simulink model "V2V"  (R2023a)
settings: Solver=FixedStepDiscrete  StartTime=0.0  StopTime=10  FixedStep=0.1  RelTol=1e-3
undefined symbols (not defined in the file): samp_time
(part 2 of 2)

== system V2V/Subsystem28/Subsystem ==
  x1 : Inport
  In2 : Inport  Port=2
  In3 : Inport  Port=3
  x2 : Inport  Port=4
  r : Inport  Port=5
  MATLAB Function : MATLAB Function  TreatAsAtomicUnit=on  SystemSampleTime=0.1
  Switch : Switch  Criteria=u2 > Threshold  SaturateOnIntegerOverflow=off  InputSameDT=off
  Out1 : Outport
  wires:
  x2/1 -> MATLAB Function/2(x2)
  x1/1 -> MATLAB Function/1(x1)
  Switch/1 -> Out1/1
  In2/1 -> Switch/1
  In3/1 -> Switch/3
  MATLAB Function/1(y) -> Switch/2
  r/1 -> MATLAB Function/3(r)

== system V2V/Subsystem30/Subsystem ==
  x1 : Inport
  In2 : Inport  Port=2
  In3 : Inport  Port=3
  x2 : Inport  Port=4
  r : Inport  Port=5
  MATLAB Function : MATLAB Function  TreatAsAtomicUnit=on  SystemSampleTime=0.1
  Switch : Switch  Criteria=u2 > Threshold  SaturateOnIntegerOverflow=off  InputSameDT=off
  Out1 : Outport
  wires:
  x2/1 -> MATLAB Function/2(x2)
  x1/1 -> MATLAB Function/1(x1)
  Switch/1 -> Out1/1
  In2/1 -> Switch/1
  In3/1 -> Switch/3
  MATLAB Function/1(y) -> Switch/2
  r/1 -> MATLAB Function/3(r)

== system V2V/Subsystem31/Subsystem ==
  x1 : Inport
  In2 : Inport  Port=2
  In3 : Inport  Port=3
  x2 : Inport  Port=4
  r : Inport  Port=5
  MATLAB Function : MATLAB Function  TreatAsAtomicUnit=on  SystemSampleTime=0.1
  Switch : Switch  Criteria=u2 > Threshold  SaturateOnIntegerOverflow=off  InputSameDT=off
  Out1 : Outport
  wires:
  x2/1 -> MATLAB Function/2(x2)
  x1/1 -> MATLAB Function/1(x1)
  Switch/1 -> Out1/1
  In2/1 -> Switch/1
  In3/1 -> Switch/3
  MATLAB Function/1(y) -> Switch/2
  r/1 -> MATLAB Function/3(r)

== system V2V/Subsystem33/Subsystem ==
  x1 : Inport
  In2 : Inport  Port=2
  In3 : Inport  Port=3
  x2 : Inport  Port=4
  r : Inport  Port=5
  MATLAB Function : MATLAB Function  TreatAsAtomicUnit=on  SystemSampleTime=0.1
  Switch : Switch  Criteria=u2 > Threshold  SaturateOnIntegerOverflow=off  InputSameDT=off
  Out1 : Outport
  wires:
  x2/1 -> MATLAB Function/2(x2)
  x1/1 -> MATLAB Function/1(x1)
  Switch/1 -> Out1/1
  In2/1 -> Switch/1
  In3/1 -> Switch/3
  MATLAB Function/1(y) -> Switch/2
  r/1 -> MATLAB Function/3(r)

== system V2V/Subsystem34/Subsystem ==
  x1 : Inport
  In2 : Inport  Port=2
  In3 : Inport  Port=3
  x2 : Inport  Port=4
  r : Inport  Port=5
  MATLAB Function : MATLAB Function  TreatAsAtomicUnit=on  SystemSampleTime=0.1
  Switch : Switch  Criteria=u2 > Threshold  SaturateOnIntegerOverflow=off  InputSameDT=off
  Out1 : Outport
  wires:
  x2/1 -> MATLAB Function/2(x2)
  x1/1 -> MATLAB Function/1(x1)
  Switch/1 -> Out1/1
  In2/1 -> Switch/1
  In3/1 -> Switch/3
  MATLAB Function/1(y) -> Switch/2
  r/1 -> MATLAB Function/3(r)

== system V2V/Subsystem36/Subsystem ==
  x1 : Inport
  In2 : Inport  Port=2
  In3 : Inport  Port=3
  x2 : Inport  Port=4
  r : Inport  Port=5
  MATLAB Function : MATLAB Function  TreatAsAtomicUnit=on  SystemSampleTime=0.1
  Switch : Switch  Criteria=u2 > Threshold  SaturateOnIntegerOverflow=off  InputSameDT=off
  Out1 : Outport
  wires:
  x2/1 -> MATLAB Function/2(x2)
  x1/1 -> MATLAB Function/1(x1)
  Switch/1 -> Out1/1
  In2/1 -> Switch/1
  In3/1 -> Switch/3
  MATLAB Function/1(y) -> Switch/2
  r/1 -> MATLAB Function/3(r)

== system V2V/Subsystem37/Subsystem ==
  x1 : Inport
  In2 : Inport  Port=2
  In3 : Inport  Port=3
  x2 : Inport  Port=4
  r : Inport  Port=5
  MATLAB Function : MATLAB Function  TreatAsAtomicUnit=on  SystemSampleTime=0.1
  Switch : Switch  Criteria=u2 > Threshold  SaturateOnIntegerOverflow=off  InputSameDT=off
  Out1 : Outport
  wires:
  x2/1 -> MATLAB Function/2(x2)
  x1/1 -> MATLAB Function/1(x1)
  Switch/1 -> Out1/1
  In2/1 -> Switch/1
  In3/1 -> Switch/3
  MATLAB Function/1(y) -> Switch/2
  r/1 -> MATLAB Function/3(r)

== system V2V/Subsystem39/Subsystem ==
  x1 : Inport
  In2 : Inport  Port=2
  In3 : Inport  Port=3
  x2 : Inport  Port=4
  r : Inport  Port=5
  MATLAB Function : MATLAB Function  TreatAsAtomicUnit=on  SystemSampleTime=0.1
  Switch : Switch  Criteria=u2 > Threshold  SaturateOnIntegerOverflow=off  InputSameDT=off
  Out1 : Outport
  wires:
  x2/1 -> MATLAB Function/2(x2)
  x1/1 -> MATLAB Function/1(x1)
  Switch/1 -> Out1/1
  In2/1 -> Switch/1
  In3/1 -> Switch/3
  MATLAB Function/1(y) -> Switch/2
  r/1 -> MATLAB Function/3(r)

== system V2V/Subsystem40/Subsystem ==
  x1 : Inport
  In2 : Inport  Port=2
  In3 : Inport  Port=3
  x2 : Inport  Port=4
  r : Inport  Port=5
  MATLAB Function : MATLAB Function  TreatAsAtomicUnit=on  SystemSampleTime=0.1
  Switch : Switch  Criteria=u2 > Threshold  SaturateOnIntegerOverflow=off  InputSameDT=off
  Out1 : Outport
  wires:
  x2/1 -> MATLAB Function/2(x2)
  x1/1 -> MATLAB Function/1(x1)
  Switch/1 -> Out1/1
  In2/1 -> Switch/1
  In3/1 -> Switch/3
  MATLAB Function/1(y) -> Switch/2
  r/1 -> MATLAB Function/3(r)

== system V2V/Subsystem42/Subsystem ==
  x1 : Inport
  In2 : Inport  Port=2
  In3 : Inport  Port=3
  x2 : Inport  Port=4
  r : Inport  Port=5
  MATLAB Function : MATLAB Function  TreatAsAtomicUnit=on  SystemSampleTime=0.1
  Switch : Switch  Criteria=u2 > Threshold  SaturateOnIntegerOverflow=off  InputSameDT=off
  Out1 : Outport
  wires:
  x2/1 -> MATLAB Function/2(x2)
  x1/1 -> MATLAB Function/1(x1)
  Switch/1 -> Out1/1
  In2/1 -> Switch/1
  In3/1 -> Switch/3
  MATLAB Function/1(y) -> Switch/2
  r/1 -> MATLAB Function/3(r)

== system V2V/Subsystem43/Subsystem ==
  x1 : Inport
  In2 : Inport  Port=2
  In3 : Inport  Port=3
  x2 : Inport  Port=4
  r : Inport  Port=5
  MATLAB Function : MATLAB Function  TreatAsAtomicUnit=on  SystemSampleTime=0.1
  Switch : Switch  Criteria=u2 > Threshold  SaturateOnIntegerOverflow=off  InputSameDT=off
  Out1 : Outport
  wires:
  x2/1 -> MATLAB Function/2(x2)
  x1/1 -> MATLAB Function/1(x1)
  Switch/1 -> Out1/1
  In2/1 -> Switch/1
  In3/1 -> Switch/3
  MATLAB Function/1(y) -> Switch/2
  r/1 -> MATLAB Function/3(r)

== system V2V/Subsystem45/Subsystem ==
  x1 : Inport
  In2 : Inport  Port=2
  In3 : Inport  Port=3
  x2 : Inport  Port=4
  r : Inport  Port=5
  MATLAB Function : MATLAB Function  TreatAsAtomicUnit=on  SystemSampleTime=0.1
  Switch : Switch  Criteria=u2 > Threshold  SaturateOnIntegerOverflow=off  InputSameDT=off
  Out1 : Outport
  wires:
  x2/1 -> MATLAB Function/2(x2)
  x1/1 -> MATLAB Function/1(x1)
  Switch/1 -> Out1/1
  In2/1 -> Switch/1
  In3/1 -> Switch/3
  MATLAB Function/1(y) -> Switch/2
  r/1 -> MATLAB Function/3(r)

== system V2V/Subsystem46/Subsystem ==
  x1 : Inport
  In2 : Inport  Port=2
  In3 : Inport  Port=3
  x2 : Inport  Port=4
  r : Inport  Port=5
  MATLAB Function : MATLAB Function  TreatAsAtomicUnit=on  SystemSampleTime=0.1
  Switch : Switch  Criteria=u2 > Threshold  SaturateOnIntegerOverflow=off  InputSameDT=off
  Out1 : Outport
  wires:
  x2/1 -> MATLAB Function/2(x2)
  x1/1 -> MATLAB Function/1(x1)
  Switch/1 -> Out1/1
  In2/1 -> Switch/1
  In3/1 -> Switch/3
  MATLAB Function/1(y) -> Switch/2
  r/1 -> MATLAB Function/3(r)

== system V2V/Subsystem48/Subsystem ==
  x1 : Inport
  In2 : Inport  Port=2
  In3 : Inport  Port=3
  x2 : Inport  Port=4
  r : Inport  Port=5
  MATLAB Function : MATLAB Function  TreatAsAtomicUnit=on  SystemSampleTime=0.1
  Switch : Switch  Criteria=u2 > Threshold  SaturateOnIntegerOverflow=off  InputSameDT=off
  Out1 : Outport
  wires:
  x2/1 -> MATLAB Function/2(x2)
  x1/1 -> MATLAB Function/1(x1)
  Switch/1 -> Out1/1
  In2/1 -> Switch/1
  In3/1 -> Switch/3
  MATLAB Function/1(y) -> Switch/2
  r/1 -> MATLAB Function/3(r)

== system V2V/Subsystem49/Subsystem ==
  x1 : Inport
  In2 : Inport  Port=2
  In3 : Inport  Port=3
  x2 : Inport  Port=4
  r : Inport  Port=5
  MATLAB Function : MATLAB Function  TreatAsAtomicUnit=on  SystemSampleTime=0.1
  Switch : Switch  Criteria=u2 > Threshold  SaturateOnIntegerOverflow=off  InputSameDT=off
  Out1 : Outport
  wires:
  x2/1 -> MATLAB Function/2(x2)
  x1/1 -> MATLAB Function/1(x1)
  Switch/1 -> Out1/1
  In2/1 -> Switch/1
  In3/1 -> Switch/3
  MATLAB Function/1(y) -> Switch/2
  r/1 -> MATLAB Function/3(r)

== system V2V/Subsystem5/Subsystem ==
  x1 : Inport
  In2 : Inport  Port=2
  In3 : Inport  Port=3
  x2 : Inport  Port=4
  r : Inport  Port=5
  MATLAB Function : MATLAB Function  TreatAsAtomicUnit=on  SystemSampleTime=0.1
  Switch : Switch  Criteria=u2 > Threshold  SaturateOnIntegerOverflow=off  InputSameDT=off
  Out1 : Outport
  wires:
  x2/1 -> MATLAB Function/2(x2)
  x1/1 -> MATLAB Function/1(x1)
  Switch/1 -> Out1/1
  In2/1 -> Switch/1
  In3/1 -> Switch/3
  MATLAB Function/1(y) -> Switch/2
  r/1 -> MATLAB Function/3(r)

== system V2V/Subsystem51/Subsystem ==
  x1 : Inport
  In2 : Inport  Port=2
  In3 : Inport  Port=3
  x2 : Inport  Port=4
  r : Inport  Port=5
  MATLAB Function : MATLAB Function  TreatAsAtomicUnit=on  SystemSampleTime=0.1
  Switch : Switch  Criteria=u2 > Threshold  SaturateOnIntegerOverflow=off  InputSameDT=off
  Out1 : Outport
  wires:
  x2/1 -> MATLAB Function/2(x2)
  x1/1 -> MATLAB Function/1(x1)
  Switch/1 -> Out1/1
  In2/1 -> Switch/1
  In3/1 -> Switch/3
  MATLAB Function/1(y) -> Switch/2
  r/1 -> MATLAB Function/3(r)

== system V2V/Subsystem52/Subsystem ==
  x1 : Inport
  In2 : Inport  Port=2
  In3 : Inport  Port=3
  x2 : Inport  Port=4
  r : Inport  Port=5
  MATLAB Function : MATLAB Function  TreatAsAtomicUnit=on  SystemSampleTime=0.1
  Switch : Switch  Criteria=u2 > Threshold  SaturateOnIntegerOverflow=off  InputSameDT=off
  Out1 : Outport
  wires:
  x2/1 -> MATLAB Function/2(x2)
  x1/1 -> MATLAB Function/1(x1)
  Switch/1 -> Out1/1
  In2/1 -> Switch/1
  In3/1 -> Switch/3
  MATLAB Function/1(y) -> Switch/2
  r/1 -> MATLAB Function/3(r)

== system V2V/Subsystem54/Subsystem ==
  x1 : Inport
  In2 : Inport  Port=2
  In3 : Inport  Port=3
  x2 : Inport  Port=4
  r : Inport  Port=5
  MATLAB Function : MATLAB Function  TreatAsAtomicUnit=on  SystemSampleTime=0.1
  Switch : Switch  Criteria=u2 > Threshold  SaturateOnIntegerOverflow=off  InputSameDT=off
  Out1 : Outport
  wires:
  x2/1 -> MATLAB Function/2(x2)
  x1/1 -> MATLAB Function/1(x1)
  Switch/1 -> Out1/1
  In2/1 -> Switch/1
  In3/1 -> Switch/3
  MATLAB Function/1(y) -> Switch/2
  r/1 -> MATLAB Function/3(r)

== system V2V/Subsystem55/Subsystem ==
  x1 : Inport
  In2 : Inport  Port=2
  In3 : Inport  Port=3
  x2 : Inport  Port=4
  r : Inport  Port=5
  MATLAB Function : MATLAB Function  TreatAsAtomicUnit=on  SystemSampleTime=0.1
  Switch : Switch  Criteria=u2 > Threshold  SaturateOnIntegerOverflow=off  InputSameDT=off
  Out1 : Outport
  wires:
  x2/1 -> MATLAB Function/2(x2)
  x1/1 -> MATLAB Function/1(x1)
  Switch/1 -> Out1/1
  In2/1 -> Switch/1
  In3/1 -> Switch/3
  MATLAB Function/1(y) -> Switch/2
  r/1 -> MATLAB Function/3(r)

== system V2V/Subsystem6/Subsystem ==
  x1 : Inport
  In2 : Inport  Port=2
  In3 : Inport  Port=3
  x2 : Inport  Port=4
  r : Inport  Port=5
  MATLAB Function : MATLAB Function  TreatAsAtomicUnit=on  SystemSampleTime=0.1
  Switch : Switch  Criteria=u2 > Threshold  SaturateOnIntegerOverflow=off  InputSameDT=off
  Out1 : Outport
  wires:
  x2/1 -> MATLAB Function/2(x2)
  x1/1 -> MATLAB Function/1(x1)
  Switch/1 -> Out1/1
  In2/1 -> Switch/1
  In3/1 -> Switch/3
  MATLAB Function/1(y) -> Switch/2
  r/1 -> MATLAB Function/3(r)

== system V2V/Subsystem7/Subsystem ==
  x1 : Inport
  In2 : Inport  Port=2
  In3 : Inport  Port=3
  x2 : Inport  Port=4
  r : Inport  Port=5
  MATLAB Function : MATLAB Function  TreatAsAtomicUnit=on  SystemSampleTime=0.1
  Switch : Switch  Criteria=u2 > Threshold  SaturateOnIntegerOverflow=off  InputSameDT=off
  Out1 : Outport
  wires:
  x2/1 -> MATLAB Function/2(x2)
  x1/1 -> MATLAB Function/1(x1)
  Switch/1 -> Out1/1
  In2/1 -> Switch/1
  In3/1 -> Switch/3
  MATLAB Function/1(y) -> Switch/2
  r/1 -> MATLAB Function/3(r)

== matlab function V2V/MATLAB Function ==
  data: delay_txL output; delay_tx2 output; delay_tx3 output; delay_tx4 output; delay_tx5 output; delay_tx6 output; delay_tx7 output; delay_tx8 output; delay_tx9 output; delay_tx10 output; delay_tx11 output; delay_tx12 output; delay_tx13 output; delay_tx14 output; delay_tx15 output; delay_tx16 output; delay_tx17 output; delay_tx18 output; delay_tx19 output; p_rx_L_2 output; p_rx_L_3 output; p_rx_L_4 output; p_rx_L_5 output; p_rx_L_6 output; p_rx_L_7 output; p_rx_L_8 output; p_rx_L_9 output; p_rx_L_10 output; p_rx_L_11 output; p_rx_L_12 output; p_rx_L_13 output; p_rx_L_14 output; p_rx_L_15 output; p_rx_L_16 output; p_rx_L_17 output; p_rx_L_18 output; p_rx_L_19 output; p_rx_L_20 output; p_rx_2_3 output; p_rx_3_4 output; p_rx_4_5 output; p_rx_5_6 output; p_rx_6_7 output; p_rx_7_8 output; p_rx_8_9 output; p_rx_9_10 output; p_rx_10_11 output; p_rx_11_12 output; p_rx_12_13 output; p_rx_13_14 output; p_rx_14_15 output; p_rx_15_16 output; p_rx_16_17 output; p_rx_17_18 output; p_rx_18_19 output; p_rx_19_20 output; data input
function [delay_txL,delay_tx2,delay_tx3,delay_tx4,delay_tx5,delay_tx6,delay_tx7,delay_tx8,delay_tx9,delay_tx10,delay_tx11,delay_tx12,delay_tx13,delay_tx14,delay_tx15,delay_tx16,delay_tx17,delay_tx18,delay_tx19,...
        p_rx_L_2,p_rx_L_3,p_rx_L_4,p_rx_L_5,p_rx_L_6,p_rx_L_7,p_rx_L_8,p_rx_L_9,p_rx_L_10,p_rx_L_11,p_rx_L_12,p_rx_L_13,p_rx_L_14,p_rx_L_15,p_rx_L_16,p_rx_L_17,p_rx_L_18,p_rx_L_19,p_rx_L_20,...
        p_rx_2_3,p_rx_3_4,p_rx_4_5,p_rx_5_6,p_rx_6_7,p_rx_7_8,p_rx_8_9,p_rx_9_10,p_rx_10_11,p_rx_11_12,p_rx_12_13,p_rx_13_14,p_rx_14_15,p_rx_15_16,p_rx_16_17,p_rx_17_18,p_rx_18_19,p_rx_19_20] = fcn(data)
delay_txL = ceil(exprnd(20));
delay_tx2 = ceil(exprnd(20));
delay_tx3 = ceil(exprnd(20));
delay_tx4 = ceil(exprnd(20));
delay_tx5 = ceil(exprnd(20));
delay_tx6 = ceil(exprnd(20));
delay_tx7 = ceil(exprnd(20));
delay_tx8 = ceil(exprnd(20));
delay_tx9 = ceil(exprnd(20));
delay_tx10 = ceil(exprnd(20));
delay_tx11 = ceil(exprnd(20));
delay_tx12 = ceil(exprnd(20));
delay_tx13 = ceil(exprnd(20));
delay_tx14 = ceil(exprnd(20));
delay_tx15 = ceil(exprnd(20));
delay_tx16 = ceil(exprnd(20));
delay_tx17 = ceil(exprnd(20));
delay_tx18 = ceil(exprnd(20));
delay_tx19 = ceil(exprnd(20));

p_rx_L_2 = rand;
p_rx_L_3 = rand;
p_rx_L_4 = rand;
p_rx_L_5 = rand;
p_rx_L_6 = rand;
p_rx_L_7 = rand;
p_rx_L_8 = rand;
p_rx_L_9 = rand;
p_rx_L_10 = rand;
p_rx_L_11 = rand;
p_rx_L_12 = rand;
p_rx_L_13 = rand;
p_rx_L_14 = rand;
p_rx_L_15 = rand;
p_rx_L_16 = rand;
p_rx_L_17 = rand;
p_rx_L_18 = rand;
p_rx_L_19 = rand;
p_rx_L_20 = rand;

p_rx_2_3 = rand;
p_rx_3_4 = rand;
p_rx_4_5 = rand;
p_rx_5_6 = rand;
p_rx_6_7 = rand;
p_rx_7_8 = rand;
p_rx_8_9 = rand;
p_rx_9_10 = rand;
p_rx_10_11 = rand;
p_rx_11_12 = rand;
p_rx_12_13 = rand;
p_rx_13_14 = rand;
p_rx_14_15 = rand;
p_rx_15_16 = rand;
p_rx_16_17 = rand;
p_rx_17_18 = rand;
p_rx_18_19 = rand;
p_rx_19_20 = rand;
end

== matlab function V2V/Subsystem10/Subsystem/MATLAB Function ==
  data: x1 input; y output; x2 input; r input
function y = fcn(x1,x2,r)
    PDR = model80211p(0.12,25,23,190,6e6,x1-x2);

    y = r < PDR;
end

== matlab function V2V/Subsystem11/Subsystem/MATLAB Function ==
  data: x1 input; y output; x2 input; r input
function y = fcn(x1,x2,r)
    PDR = model80211p(0.12,25,23,190,6e6,x1-x2);

    y = r < PDR;
end

== matlab function V2V/Subsystem12/Subsystem/MATLAB Function ==
  data: x1 input; y output; x2 input; r input
function y = fcn(x1,x2,r)
    PDR = model80211p(0.12,25,23,190,6e6,x1-x2);

    y = r < PDR;
end

== matlab function V2V/Subsystem5/Subsystem/MATLAB Function ==
  data: x1 input; y output; x2 input; r input
function y = fcn(x1,x2,r)
    PDR = model80211p(0.12,25,23,190,6e6,x1-x2);

    y = r < PDR;
end

== matlab function V2V/Subsystem13/Subsystem/MATLAB Function ==
  data: x1 input; y output; x2 input; r input
function y = fcn(x1,x2,r)
    PDR = model80211p(0.12,25,23,190,6e6,x1-x2);

    y = r < PDR;
end

== matlab function V2V/Subsystem15/Subsystem/MATLAB Function ==
  data: x1 input; y output; x2 input; r input
function y = fcn(x1,x2,r)
    PDR = model80211p(0.12,25,23,190,6e6,x1-x2);

    y = r < PDR;
end

== matlab function V2V/Subsystem16/Subsystem/MATLAB Function ==
  data: x1 input; y output; x2 input; r input
function y = fcn(x1,x2,r)
    PDR = model80211p(0.12,25,23,190,6e6,x1-x2);

    y = r < PDR;
end

== matlab function V2V/Subsystem18/Subsystem/MATLAB Function ==
  data: x1 input; y output; x2 input; r input
function y = fcn(x1,x2,r)
    PDR = model80211p(0.12,25,23,190,6e6,x1-x2);

    y = r < PDR;
end

== matlab function V2V/Subsystem19/Subsystem/MATLAB Function ==
  data: x1 input; y output; x2 input; r input
function y = fcn(x1,x2,r)
    PDR = model80211p(0.12,25,23,190,6e6,x1-x2);

    y = r < PDR;
end

== matlab function V2V/Subsystem21/Subsystem/MATLAB Function ==
  data: x1 input; y output; x2 input; r input
function y = fcn(x1,x2,r)
    PDR = model80211p(0.12,25,23,190,6e6,x1-x2);

    y = r < PDR;
end

== matlab function V2V/Subsystem22/Subsystem/MATLAB Function ==
  data: x1 input; y output; x2 input; r input
function y = fcn(x1,x2,r)
    PDR = model80211p(0.12,25,23,190,6e6,x1-x2);

    y = r < PDR;
end

== matlab function V2V/Subsystem24/Subsystem/MATLAB Function ==
  data: x1 input; y output; x2 input; r input
function y = fcn(x1,x2,r)
    PDR = model80211p(0.12,25,23,190,6e6,x1-x2);

    y = r < PDR;
end

== matlab function V2V/Subsystem25/Subsystem/MATLAB Function ==
  data: x1 input; y output; x2 input; r input
function y = fcn(x1,x2,r)
    PDR = model80211p(0.12,25,23,190,6e6,x1-x2);

    y = r < PDR;
end

== matlab function V2V/Subsystem27/Subsystem/MATLAB Function ==
  data: x1 input; y output; x2 input; r input
function y = fcn(x1,x2,r)
    PDR = model80211p(0.12,25,23,190,6e6,x1-x2);

    y = r < PDR;
end

== matlab function V2V/Subsystem28/Subsystem/MATLAB Function ==
  data: x1 input; y output; x2 input; r input
function y = fcn(x1,x2,r)
    PDR = model80211p(0.12,25,23,190,6e6,x1-x2);

    y = r < PDR;
end

== matlab function V2V/Subsystem30/Subsystem/MATLAB Function ==
  data: x1 input; y output; x2 input; r input
function y = fcn(x1,x2,r)
    PDR = model80211p(0.12,25,23,190,6e6,x1-x2);

    y = r < PDR;
end

== matlab function V2V/Subsystem31/Subsystem/MATLAB Function ==
  data: x1 input; y output; x2 input; r input
function y = fcn(x1,x2,r)
    PDR = model80211p(0.12,25,23,190,6e6,x1-x2);

    y = r < PDR;
end

== matlab function V2V/Subsystem33/Subsystem/MATLAB Function ==
  data: x1 input; y output; x2 input; r input
function y = fcn(x1,x2,r)
    PDR = model80211p(0.12,25,23,190,6e6,x1-x2);

    y = r < PDR;
end

== matlab function V2V/Subsystem34/Subsystem/MATLAB Function ==
  data: x1 input; y output; x2 input; r input
function y = fcn(x1,x2,r)
    PDR = model80211p(0.12,25,23,190,6e6,x1-x2);

    y = r < PDR;
end

== matlab function V2V/Subsystem36/Subsystem/MATLAB Function ==
  data: x1 input; y output; x2 input; r input
function y = fcn(x1,x2,r)
    PDR = model80211p(0.12,25,23,190,6e6,x1-x2);

    y = r < PDR;
end

== matlab function V2V/Subsystem37/Subsystem/MATLAB Function ==
  data: x1 input; y output; x2 input; r input
function y = fcn(x1,x2,r)
    PDR = model80211p(0.12,25,23,190,6e6,x1-x2);

    y = r < PDR;
end

== matlab function V2V/Subsystem39/Subsystem/MATLAB Function ==
  data: x1 input; y output; x2 input; r input
function y = fcn(x1,x2,r)
    PDR = model80211p(0.12,25,23,190,6e6,x1-x2);

    y = r < PDR;
end

== matlab function V2V/Subsystem40/Subsystem/MATLAB Function ==
  data: x1 input; y output; x2 input; r input
function y = fcn(x1,x2,r)
    PDR = model80211p(0.12,25,23,190,6e6,x1-x2);

    y = r < PDR;
end

== matlab function V2V/Subsystem42/Subsystem/MATLAB Function ==
  data: x1 input; y output; x2 input; r input
function y = fcn(x1,x2,r)
    PDR = model80211p(0.12,25,23,190,6e6,x1-x2);

    y = r < PDR;
end

== matlab function V2V/Subsystem43/Subsystem/MATLAB Function ==
  data: x1 input; y output; x2 input; r input
function y = fcn(x1,x2,r)
    PDR = model80211p(0.12,25,23,190,6e6,x1-x2);

    y = r < PDR;
end

== matlab function V2V/Subsystem45/Subsystem/MATLAB Function ==
  data: x1 input; y output; x2 input; r input
function y = fcn(x1,x2,r)
    PDR = model80211p(0.12,25,23,190,6e6,x1-x2);

    y = r < PDR;
end

== matlab function V2V/Subsystem46/Subsystem/MATLAB Function ==
  data: x1 input; y output; x2 input; r input
function y = fcn(x1,x2,r)
    PDR = model80211p(0.12,25,23,190,6e6,x1-x2);

    y = r < PDR;
end

== matlab function V2V/Subsystem48/Subsystem/MATLAB Function ==
  data: x1 input; y output; x2 input; r input
function y = fcn(x1,x2,r)
    PDR = model80211p(0.12,25,23,190,6e6,x1-x2);

    y = r < PDR;
end

== matlab function V2V/Subsystem49/Subsystem/MATLAB Function ==
  data: x1 input; y output; x2 input; r input
function y = fcn(x1,x2,r)
    PDR = model80211p(0.12,25,23,190,6e6,x1-x2);

    y = r < PDR;
end

== matlab function V2V/Subsystem51/Subsystem/MATLAB Function ==
  data: x1 input; y output; x2 input; r input
function y = fcn(x1,x2,r)
    PDR = model80211p(0.12,25,23,190,6e6,x1-x2);

    y = r < PDR;
end

== matlab function V2V/Subsystem52/Subsystem/MATLAB Function ==
  data: x1 input; y output; x2 input; r input
function y = fcn(x1,x2,r)
    PDR = model80211p(0.12,25,23,190,6e6,x1-x2);

    y = r < PDR;
end

== matlab function V2V/Subsystem54/Subsystem/MATLAB Function ==
  data: x1 input; y output; x2 input; r input
function y = fcn(x1,x2,r)
    PDR = model80211p(0.12,25,23,190,6e6,x1-x2);

    y = r < PDR;
end

== matlab function V2V/Subsystem55/Subsystem/MATLAB Function ==
  data: x1 input; y output; x2 input; r input
function y = fcn(x1,x2,r)
    PDR = model80211p(0.12,25,23,190,6e6,x1-x2);

    y = r < PDR;
end

== matlab function V2V/Subsystem1/Subsystem/MATLAB Function ==
  data: x1 input; y output; x2 input; r input
function y = fcn(x1,x2,r)
    PDR = model80211p(0.12,25,23,190,6e6,x1-x2);

    y = r < PDR;
end

== matlab function V2V/Subsystem2/Subsystem/MATLAB Function ==
  data: x1 input; y output; x2 input; r input
function y = fcn(x1,x2,r)
    PDR = model80211p(0.12,25,23,190,6e6,x1-x2);

    y = r < PDR;
end

== matlab function V2V/Subsystem6/Subsystem/MATLAB Function ==
  data: x1 input; y output; x2 input; r input
function y = fcn(x1,x2,r)
    PDR = model80211p(0.12,25,23,190,6e6,x1-x2);

    y = r < PDR;
end

== matlab function V2V/Subsystem7/Subsystem/MATLAB Function ==
  data: x1 input; y output; x2 input; r input
function y = fcn(x1,x2,r)
    PDR = model80211p(0.12,25,23,190,6e6,x1-x2);

    y = r < PDR;
end
